simulink model "actuactor_model_2023a"  (R2023a)
settings: Solver=FixedStepAuto  StartTime=0.0  StopTime=stop_time  FixedStep=timestep  RelTol=1e-3
values from neighbouring files (symbols this model uses):
  average_thruster = mean( y2( OS( Step_test_open_signal+10):OS(end) ) )    [thrusterDataProcess.m]
  dp = 0.4113    [thrusterDataProcess.m]
  lag_time = 0.094    [thrusterDataProcess.m]
  wn = 49.2375    [thrusterDataProcess.m]
settings Model: Creator=s3928  LastModifiedBy=s3928

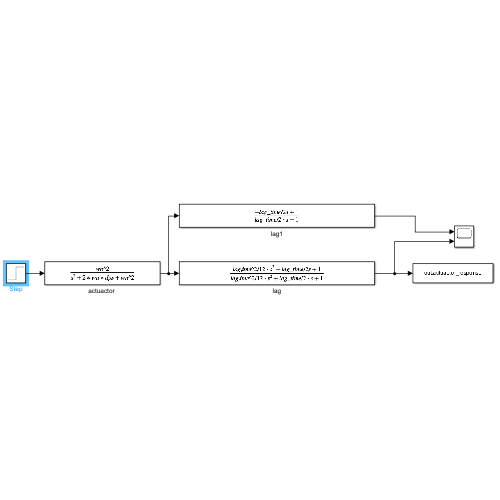
[thumbnail: Simulink's stored preview of the top-level diagram]
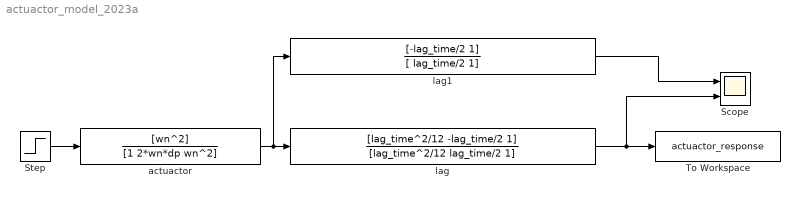
== system actuactor_model_2023a ==
  Scope : Scope  NumInputPorts=2
  Step : Step  Time=0  After=average_thruster  SampleTime=0
  To Workspace : ToWorkspace  VariableName=actuactor_response  SaveFormat=Timeseries  SampleTime=-1
  "actuactor " : TransferFcn  Numerator=[wn^2]  Denominator=[1 2*wn*dp wn^2]
  lag : TransferFcn  Numerator=[lag_time^2/12 -lag_time/2 1]  Denominator=[lag_time^2/12 lag_time/2 1]
  lag1 : TransferFcn  Numerator=[-lag_time/2 1]  Denominator=[ lag_time/2 1]
  wires:
  Step/1 -> "actuactor "/1
  "actuactor "/1 -> lag1/1, lag/1
  lag/1 -> Scope/2, To Workspace/1
  lag1/1 -> Scope/1
